simulink model "PID_Controller"  (R2024b)
settings: Solver=VariableStepAuto  StartTime=0.0  StopTime=10.0  RelTol=1e-3
undefined symbols (not defined in the file or in its folder): Kd, Kp
settings Model: Creator=jakub  LastModifiedBy=jakub

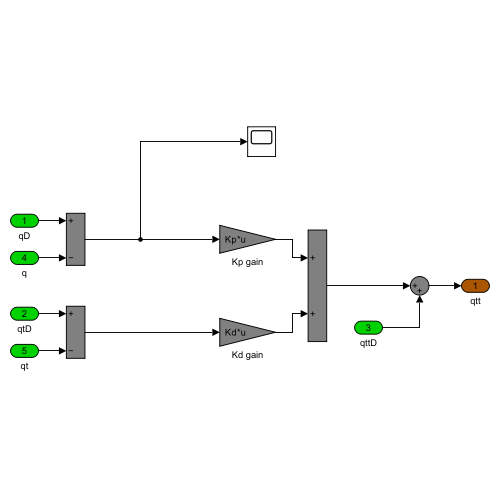
[thumbnail: Simulink's stored preview of the top-level diagram]
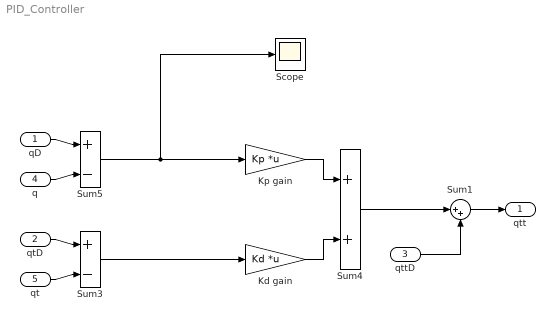
== system PID_Controller ==
  qD : Inport  OutDataTypeStr=double  Unit=rad  PortDimensions=[2 1]  SampleTime=0
  qtD : Inport  Port=2  OutDataTypeStr=double  Unit=rad/s  PortDimensions=[2 1]  SampleTime=0
  qttD : Inport  Port=3  OutDataTypeStr=double  Unit=rad/s^2  PortDimensions=[2 1]  SampleTime=0
  q : Inport  Port=4  OutDataTypeStr=double  Unit=rad  PortDimensions=[2 1]  SampleTime=0
  qt : Inport  Port=5  OutDataTypeStr=double  Unit=rad/s  PortDimensions=[2 1]  SampleTime=0
  Kd gain : Gain  Gain=Kd  Multiplication=Matrix(K*u)  OutDataTypeStr=double
  Kp gain : Gain  Gain=Kp  Multiplication=Matrix(K*u)  OutDataTypeStr=double
  Scope : Scope
  Sum1 : Sum  Inputs=|++  OutDataTypeStr=double
  Sum3 : Sum  Inputs=+|-  OutDataTypeStr=double
  Sum4 : Sum  OutDataTypeStr=double
  Sum5 : Sum  Inputs=+|-  OutDataTypeStr=double
  qtt : Outport  OutDataTypeStr=double  Unit=rad/s^2  PortDimensions=[2 1]  SampleTime=0
  wires:
  qD/1 -> Sum5/1
  Sum1/1 -> qtt/1
  qtD/1 -> Sum3/1
  Sum4/1 -> Sum1/1
  qttD/1 -> Sum1/2
  q/1 -> Sum5/2
  qt/1 -> Sum3/2
  Kd gain/1 -> Sum4/2
  Kp gain/1 -> Sum4/1
  Sum3/1 -> Kd gain/1
  Sum5/1 -> Scope/1, Kp gain/1
